simulink model "SOLARPV_BATTERY_HYBRID"  (R2023b)
settings: Solver=ode23t  StartTime=0.0  StopTime=5  FixedStep=1e-5  MaxStep=1e-4  RelTol=10e-4  EnableMultiTasking=on
undefined symbols (not defined in the file): Ion, Lithium
libraries: spsFirstOrderFilterLib x8, spsSeriesRLCBranchLib x7, simulink x7, spsCurrentMeasurementLib x4, spsPWMGeneratorDCDCLib x3, spsVoltageMeasurementLib x3, spsIGBTDiodeLib x3, slpidlib x2, spsGroundLib x2, spsPermanentMagnetSynchronousMachineLib x1, spsUniversalBridgeLib x1, spsBatteryLib x1
settings Model: Creator=Administrator  LastModifiedBy=NADIN
settings SolverCC: ZeroCrossControl=DisableAll  AlgebraicLoopSolver=TrustRegion
settings DataIOCC: LimitDataPoints=on  SaveFormat=Array  SignalLoggingSaveFormat=ModelDataLogs  ReturnWorkspaceOutputs=off
settings OptimizationCC: ExpressionDepthLimit=2147483647  LifeSpan=inf
settings DebuggingCC: UnderspecifiedInitializationDetection=Classic  MergeDetectMultiDrivingBlocksExec=none  SolverPrmCheckMsg=warning  FcnCallInpInsideContextMsg=warning  UnconnectedInputMsg=warning  UnconnectedOutputMsg=warning  UnconnectedLineMsg=warning  StateNameClashWarn=warning  SFUnexpectedBacktrackingDiag=warning  SFNoUnconditionalDefaultTransitionDiag=warning  SFExecutionAtInitializationDiag=none  ArithmeticOperatorsInVariantConditions=warning
settings HardwareCC: ProdBitPerPointer=32  ProdBitPerSizeT=32  ProdBitPerPtrDiffT=32  ProdLargestAtomicFloat=None  ProdIntDivRoundTo=Undefined  ProdEndianess=Unspecified  ProdWordSize=32  ProdHWDeviceType=32-bit Generic
settings ModelReferenceCC: EnableRefExpFcnMdlSchedulingChecks=on  PropagateSignalLabelsOutOfModel=off
settings SFSimCC: SimUseLocalCustomCode=off  CustomCodeUndefinedFunction=UseInterfaceOnly
settings RTWCC: RTWUseLocalCustomCode=off
settings CodeAppCC: StateflowObjectComments=on
settings GRTTargetCC: TargetLangStandard=C89/C90 (ANSI)  CombineOutputUpdateFcns=off  GRTInterface=on
settings ConfigComp: CovMetricSettings=dw  CovSaveCumulativeToWorkspaceVar=on  CovSaveSingleToWorkspaceVar=on  CovExternalEMLEnable=off
settings SimscapeCC: SimscapeNormalizeSystem=off

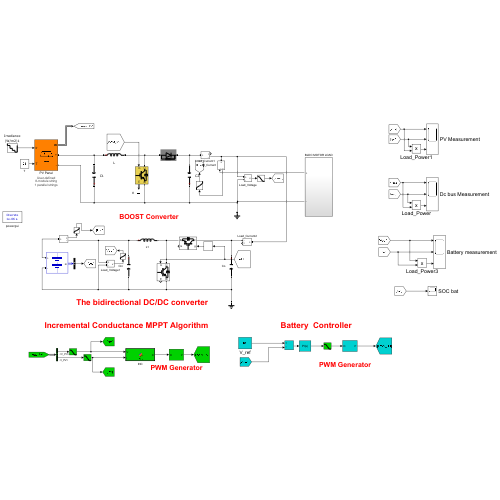
[thumbnail: Simulink's stored preview of the top-level diagram]
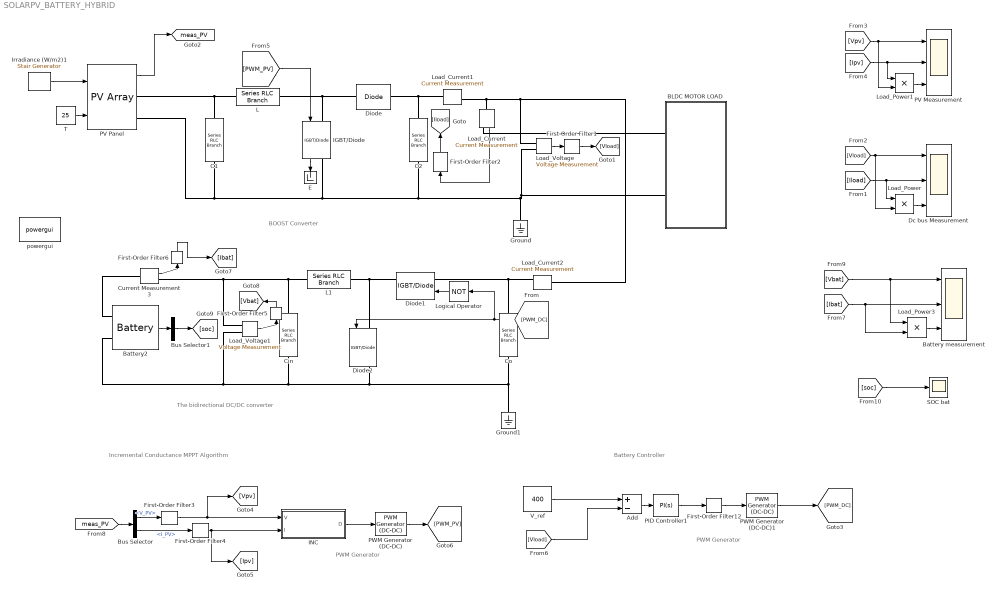
== system SOLARPV_BATTERY_HYBRID ==
  note: BOOST Converter
  note: Incremental Conductance MPPT Algorithm
  note: PWM Generator
  note: The bidirectional DC/DC converter
  note: PWM Generator
  note: Battery Controller
  Add : Sum  Inputs=+-
  BLDC MOTOR LOAD : Subsystem
  Battery measurement : Scope  NumInputPorts=3
  Battery2 : spsBatteryLib/Battery  BatType=Lithium-Ion  ShowTempParam=off  ThermalPreset=no  ShowAgeParam=off  NomV=12*20  NomQ=48  SOC=50  Batt_Tr=0.0001  PresetModel=on  MaxQ=48  MinV=180  FullV=279.3569  Dis_rate=20.8696  R=0.05  Normal_OP=43.4087  expZone="[259.2926      2.358261]"  current=[1.5 3]  Units=Ampere-hour  Tci=20  NomT=20  T2=-30  MaxQ2=4.8  FullV2=7.1  Normal_OP2=5.72  expZone2="[6.58  1]"  Rca=0.6  ti=1000  Dp=0  Neq0=0  Tsim=1e6  Ta1=25  Qeol=5.4*0.9  Reol=0.013333*1.2  Char_age=[2.3478, 3]  Dis_age=[2.3478, 10]  N1=1500  N2=10500  N3=1000  N4=1400  Ta2=45  N5=950
      settings: LibrarySourceBlock=electricdrivelib/Extra Sources/Battery
  Bus Selector : BusSelector  OutputSignals=V_PV,I_PV
  Bus Selector1 : BusSelector  OutputSignals=SOC (%)  OutputAsBus=on
  C1 : spsSeriesRLCBranchLib/Series RLC Branch  LConnTagsString=__new0  RConnTagsString=__new0  BranchType=C  Resistance=1  Inductance=1e-3  SetiL0=off  InitialCurrent=0  Capacitance=4.8250e-05  Setx0=off  InitialVoltage=0  Measurements=None
  C2 : spsSeriesRLCBranchLib/Series RLC Branch  LConnTagsString=__new0  RConnTagsString=__new0  BranchType=C  Resistance=1  Inductance=1e-3  SetiL0=off  InitialCurrent=0  Capacitance=4.8250e-05  Setx0=off  InitialVoltage=0  Measurements=None
  Cin : spsSeriesRLCBranchLib/Series RLC Branch  LConnTagsString=__new0  RConnTagsString=__new0  BranchType=C  Resistance=1  Inductance=3e-3  SetiL0=off  InitialCurrent=0  Capacitance=4.8250e-05  Setx0=off  InitialVoltage=0  Measurements=None
  Co : spsSeriesRLCBranchLib/Series RLC Branch  LConnTagsString=__new0  RConnTagsString=__new0  BranchType=C  Resistance=1  Inductance=3e-3  SetiL0=off  InitialCurrent=0  Capacitance=4.8250e-05  Setx0=off  InitialVoltage=0  Measurements=None
  Current Measurement3 : spsCurrentMeasurementLib/Current Measurement  PhasorSimulation=off  OutputType=Complex  PSBequivalent=0
  Dc bus Measurement : Scope  NumInputPorts=3
  Diode : spsDiodeLib/Diode  Ron=0.001  Lon=0  Vf=0.8  IC=0  UseSnubber=off  Rs=500  Cs=250e-9  Measurements=off
  Diode1 : spsIGBTDiodeLib/IGBT//Diode  Ron=1e-3  Rs=1e5  Cs=inf  Measurements=on
  Diode2 : spsIGBTDiodeLib/IGBT//Diode  Ron=1e-3  Rs=1e5  Cs=inf  Measurements=on
  E : Terminator
  First-Order Filter{1..6,12} (7 alike) : spsFirstOrderFilterLib/First-Order Filter  FilterType=Lowpass  Tc=10e-3  Ts=0  Initialize=on  Vac_Init=[0, 0, 60]  Vdc_Init=0  PlotResponse=off  FreqRange="[0,  200,  1]"
  Ground : spsGroundLib/Ground  LConnTagsString=a
  Ground1 : spsGroundLib/Ground  LConnTagsString=a
  IGBT/Diode : spsIGBTDiodeLib/IGBT//Diode  Ron=1e-3  Rs=1e5  Cs=inf  Measurements=on
  INC : MATLAB Function  TreatAsAtomicUnit=on
  Irradiance (W/m2)1 : spsStairGeneratorLib/Stair Generator  t=[0, 0.3, 0.6,0.9, 1.2,1.5]*(1/0.3)  e=[1, 0.8, 0.5, 0.3, 0.1,0.8]*1000  Ts=0.0001
  L : spsSeriesRLCBranchLib/Series RLC Branch  LConnTagsString=__new0  RConnTagsString=__new0  BranchType=L  Resistance=1  Inductance=0.1164  SetiL0=off  InitialCurrent=0  Capacitance=1e-6  Setx0=off  InitialVoltage=0  Measurements=None
  L1 : spsSeriesRLCBranchLib/Series RLC Branch  LConnTagsString=__new0  RConnTagsString=__new0  BranchType=L  Resistance=.25  Inductance=0.1164  SetiL0=off  InitialCurrent=0  Capacitance=1e-6  Setx0=off  InitialVoltage=0  Measurements=None
  Load_Current : spsCurrentMeasurementLib/Current Measurement  PhasorSimulation=off  OutputType=Complex  PSBequivalent=0
  Load_Current1 : spsCurrentMeasurementLib/Current Measurement  PhasorSimulation=off  OutputType=Complex  PSBequivalent=0
  Load_Current2 : spsCurrentMeasurementLib/Current Measurement  PhasorSimulation=off  OutputType=Complex  PSBequivalent=0
  Load_Power : Product  RndMeth=Zero
  Load_Power1 : Product  RndMeth=Zero
  Load_Power3 : Product  RndMeth=Zero
  Load_Voltage : spsVoltageMeasurementLib/Voltage Measurement  PhasorSimulation=off  OutputType=Complex  PSBequivalent=0
  Load_Voltage1 : spsVoltageMeasurementLib/Voltage Measurement  PhasorSimulation=off  OutputType=Complex  PSBequivalent=0
  Logical Operator : Logic  Operator=NOT  AllPortsSameDT=off  OutDataTypeStr=boolean
  PID Controller1 : slpidlib/PID Controller  Controller=PI  Form=Parallel  TimeDomain=Continuous-time  UseExternalTs=off  SampleTime=-1  IntegratorMethod=Forward Euler  FilterMethod=Forward Euler  ControllerParametersSource=internal  P=0.0001  I=0.02  UseKiTs=off  D=0  N=100  UseFilter=on  TunerSelectOption=Transfer Function Based (PID Tuner App)  InitialConditionSource=internal  InitialConditionForIntegrator=0  InitialConditionForFilter=0  DifferentiatorICPrevScaledInput=0  ExternalReset=none  TrackingMode=off  Kt=1  LimitOutput=off  SatLimitsSource=internal  UpperSaturationLimit=inf  LowerSaturationLimit=-inf  LinearizeAsGain=on  AntiWindupMode=none  Kb=1  LimitIntegrator=off  UpperIntegratorSaturationLimit=inf  LowerIntegratorSaturationLimit=-inf  POutMin=[]  POutMax=[]  IOutMin=[]  IOutMax=[]  DOutMin=[]  DOutMax=[]  NOutMin=[]  NOutMax=[]  SumOutMin=[]  SumOutMax=[]  SaturationOutMin=[]  SaturationOutMax=[]  PParamMin=[]  PParamMax=[]  IParamMin=[]  IParamMax=[]  DParamMin=[]  DParamMax=[]  NParamMin=[]  NParamMax=[]  KbParamMin=[]  KbParamMax=[]  KtParamMin=[]  KtParamMax=[]  KbOutMin=[]  KbOutMax=[]  KtOutMin=[]  KtOutMax=[]  IntegratorOutMin=[]  IntegratorOutMax=[]  FilterOutMin=[]  FilterOutMax=[]  SumI1OutMin=[]  SumI1OutMax=[]  SumI2OutMin=[]  SumI2OutMax=[]  SumI3OutMin=[]  SumI3OutMax=[]  SumI4OutMin=[]  SumI4OutMax=[]  SumDOutMin=[]  SumDOutMax=[]  DifferentiatorOutMin=[]  DifferentiatorOutMax=[]  FilterDiffOutCoefMin=[]  FilterDiffOutCoefMax=[]  ReciprocalOutMin=[]  ReciprocalOutMax=[]  SumDenOutMin=[]  SumDenOutMax=[]  SumNumOutMin=[]  SumNumOutMax=[]  DivideOutMin=[]  DivideOutMax=[]  UdiffTsProdOutMin=[]  UdiffTsProdOutMax=[]  NTsProdOutMin=[]  NTsProdOutMax=[]  UintegralTsProdOutMin=[]  UintegralTsProdOutMax=[]  UngainTsProdOutMin=[]  UngainTsProdOutMax=[]  ClampingZeroOutDataTypeStr=Inherit: Inherit via back propagation  ClampingZeroOutMin=[]  ClampingZeroOutMax=[]  FilterDenConstantOutDataTypeStr=Inherit: Inherit via back propagation  FilterDenConstantOutMin=[]  FilterDenConstantOutMax=[]  PCopyOutDataTypeStr=Inherit: Inherit via back propagation  PCopyOutMin=[]  PCopyOutMax=[]  NCopyOutDataTypeStr=Inherit: Inherit via back propagation  NCopyOutMin=[]  NCopyOutMax=[]  IntegratorContinuousStateAttributes=''  IntegratorStateMustResolveToSignalObject=off  IntegratorRTWStateStorageClass=Auto  FilterContinuousStateAttributes=''  FilterStateMustResolveToSignalObject=off  FilterRTWStateStorageClass=Auto  ParallelPVariant=InternalParameters  IdealPVariant=Disabled  IVariant=InternalParameters  DVariant=Disabled  IntegratorVariant=Continuous  SatVariant=Disabled  AWVariant=Passthrough  PCopyVariant=Disabled  TRVariant=Disabled  FdbkBlocksVariant=Forward  IdealPFdbkVariant=Disabled  SatFdbkVariant=Disabled  DerivativeFilterVariant=Disabled  NVariant=Disabled  NCopyVariant=Disabled_SignalSpec  FilterICVariant=Disabled  IntegratorICVariant=InternalICs  ExternalResetVariant=Disabled  TRSumVariant=Passthrough  SumFdbkVariant=Disabled  SumVariant=Sum_PI  TsampFilterVariant=InternalTs  TsampNgainVariant=Passthrough  TsampIntegralVariant=Disabled_SignalSpec  ExternalSaturationOutDataTypeStr=Inherit: Same as second input
  PV Measurement : Scope  NumInputPorts=3
  PV Panel : spsPVArrayLib/PV Array  Npar=1  Nser=8  PlotType=array @ 25 deg.C & specified irradiances  S_vec="[ 1000 800  600  400 ]"  Temp_C_vec="[ 45 25  ]"  ModuleName=User-defined  PlotWhenSelected=off  Pm=250.205  Ncell=60  Voc=37.3  Isc=8.66  Vm=30.7  Im=8.15  beta_Voc_pc=-0.36901  alpha_Isc_pc=0.086998  beta_Voc=-0.13764  alpha_Isc=0.007534  IL=8.7062  I0=4.1579e-10  nI=1.0189  Rsh=240.6015  Rs=0.23732  RobustModel=off  RobustCellTemperature=313.3991  BAL=on  Tc=1e-6  Tfilter=1e-5
      settings: AttributesFormatString=|
      | %<ModuleName>
      | %<Nser>-module string
      | %<Npar> parallel strings
  PWM Generator (DC-DC) : spsPWMGeneratorDCDCLib/PWM Generator (DC-DC)  Fsw=10000  Ts=0
  PWM Generator (DC-DC)1 : spsPWMGeneratorDCDCLib/PWM Generator (DC-DC)  Fsw=10000  Ts=0
  SOC bat : Scope
  T : Constant  Value=25
  V_ref : Constant  Value=400
  powergui : sps_lib/powergui  Priority=1  SimulationMode=Discrete  SampleTime=1e-6  frequency=60  Iterations=50  frequencyindice=0  Pbase=100e6  ErrMax=1e-4  UnitsV=kV  UnitsW=MW  buscounter=0  FunctionMessages=off  echomessages=off  EnableUseOfTLC=off  CurrentSourceSwitches=off  DisableSnubberDevices=off  DisableRonSwitches=off  DisableVfSwitches=off  DisplayEquations=off  AutomaticDiscreteSolvers=off  SolverType=Tustin/Backward Euler (TBE)  Interpol=off  ExternalGateDelay=off  methode=off  Ts=100  x0status=blocks  SPID=on  SwTol=0  HookPort=off  NonlinearTolerance=1e-4  nMaxIteration=100  ContinueOnMaxIteration=off  RestoreLinks=warning  ResistiveCurrentMeasurement=off  Frange=[0:2:500]  Ylog=off  Xlog=on  ShowGrid=off  save=off  variable=ZData  structure=0  ZoomFFT=off  StartTime=0.0  cycles=1  DisplayStyle=1  fundamental=60  FreqAxis=off  MaxFrequency=1000  frequencyindicesteady=1  RmsSteady=1  display=off
  tag scope: meas_PV=global
  wires:
  T/1 -> PV Panel/2
  IGBT/Diode/1 -> E/1
  PV Panel/1 -> [meas_PV]
  [meas_PV] -> Bus Selector/1
  Bus Selector/2 -> First-Order Filter4/1  "<I_PV>"
  Bus Selector/1 -> First-Order Filter3/1  "<V_PV>"
  INC/1(D) -> PWM Generator (DC-DC)/1
  V_ref/1 -> Add/1
  [Vload] -> Add/2
  Load_Voltage/1 -> First-Order Filter1/1
  Load_Current/1 -> First-Order Filter2/1
  First-Order Filter3/1 -> [Vpv], INC/1(V)
  First-Order Filter4/1 -> [Ipv], INC/2(I)
  Battery2/1 -> Bus Selector1/1
  Logical Operator/1 -> Diode1/1
  First-Order Filter2/1 -> [Iload]
  First-Order Filter1/1 -> [Vload]
  PWM Generator (DC-DC)/1 -> [PWM_PV]
  [PWM_PV] -> IGBT/Diode/1
  PWM Generator (DC-DC)1/1 -> [PWM_DC]
  [PWM_DC] -> Logical Operator/1, Diode2/1
  Current Measurement3/1 -> First-Order Filter6/1
  Load_Voltage1/1 -> First-Order Filter5/1
  Bus Selector1/1 -> [soc]
  [Vpv] -> Load_Power1/2, PV Measurement/1
  [Ipv] -> Load_Power1/1, PV Measurement/2
  Load_Power1/1 -> PV Measurement/3
  [Ibat] -> Load_Power3/2, Battery measurement/2
  [Vbat] -> Load_Power3/1, Battery measurement/1
  First-Order Filter6/1 -> [Ibat]
  First-Order Filter5/1 -> [Vbat]
  [Vload] -> Load_Power/2, Dc bus Measurement/1
  [Iload] -> Load_Power/1, Dc bus Measurement/2
  Load_Power/1 -> Dc bus Measurement/3
  [soc] -> SOC bat/1
  Load_Power3/1 -> Battery measurement/3
  PID Controller1/1 -> First-Order Filter12/1
  Add/1 -> PID Controller1/1
  First-Order Filter12/1 -> PWM Generator (DC-DC)1/1
  Irradiance (W/m2)1/1 -> PV Panel/1
  connections:
  L/LConn1 -- PV Panel/RConn1 -- C1/RConn1
  L/RConn1 -- Diode/LConn1 -- IGBT/Diode/LConn1
  Load_Voltage/LConn2 -- PV Panel/RConn2 -- C1/LConn1 -- IGBT/Diode/RConn1 -- C2/LConn1 -- Ground/LConn1 -- BLDC MOTOR LOAD/RConn2
  Diode/RConn1 -- Load_Current1/LConn1 -- C2/RConn1
  Current Measurement3/LConn1 -- Battery2/LConn1
  Load_Voltage1/LConn1 -- Current Measurement3/RConn1 -- L1/LConn1 -- Cin/LConn1
  Diode2/LConn1 -- Diode1/RConn1 -- L1/RConn1
  BLDC MOTOR LOAD/RConn1 -- Load_Current/RConn1
  Co/RConn1 -- Ground1/LConn1 -- Load_Voltage1/LConn2 -- Battery2/LConn2 -- Cin/RConn1 -- Diode2/RConn1
  Co/LConn1 -- Load_Current2/RConn1 -- Diode1/LConn1
  Load_Current1/RConn1 -- Load_Current2/LConn1 -- Load_Voltage/LConn1 -- Load_Current/LConn1

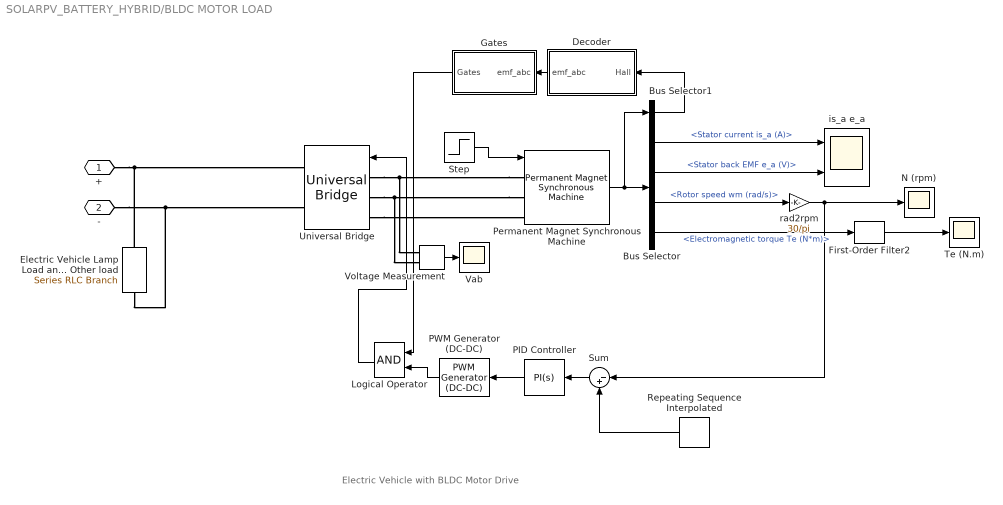
== system SOLARPV_BATTERY_HYBRID/BLDC MOTOR LOAD ==
  note: Electric Vehicle with BLDC Motor Drive
  Bus Selector : BusSelector  OutputSignals=Stator current is_a (A),Stator back EMF e_a (V),Rotor speed wm (rad/s),Electromagnetic torque Te (N*m)
  Bus Selector1 : BusSelector  OutputSignals=Hall effect signal h_a,Hall effect signal h_b,Hall effect signal h_c  OutputAsBus=on
  Decoder : Subsystem
  Electric Vehicle Lamp Load and Other load : spsSeriesRLCBranchLib/Series RLC Branch  LConnTagsString=__new0  RConnTagsString=__new0  BranchType=R  Resistance=400*400/1000  Inductance=1e-3  SetiL0=off  InitialCurrent=0  Capacitance=1e-6  Setx0=off  InitialVoltage=0  Measurements=None
  First-Order Filter2 : spsFirstOrderFilterLib/First-Order Filter  FilterType=Lowpass  Tc=10e-3  Ts=0  Initialize=on  Vac_Init=[0, 0, 60]  Vdc_Init=0  PlotResponse=off  FreqRange="[0,  200,  1]"
  Gates : Subsystem
  Logical Operator : Logic  AllPortsSameDT=off  OutDataTypeStr=boolean
  N (rpm) : Scope
  PID Controller : slpidlib/PID Controller  Controller=PI  Form=Parallel  TimeDomain=Continuous-time  UseExternalTs=off  SampleTime=-1  IntegratorMethod=Forward Euler  FilterMethod=Forward Euler  ControllerParametersSource=internal  P=1  I=1  UseKiTs=off  D=0  N=100  UseFilter=on  TunerSelectOption=Transfer Function Based (PID Tuner App)  InitialConditionSource=internal  InitialConditionForIntegrator=0  InitialConditionForFilter=0  DifferentiatorICPrevScaledInput=0  ExternalReset=none  TrackingMode=off  Kt=1  LimitOutput=off  SatLimitsSource=internal  UpperSaturationLimit=inf  LowerSaturationLimit=-inf  LinearizeAsGain=on  AntiWindupMode=none  Kb=1  LimitIntegrator=off  UpperIntegratorSaturationLimit=inf  LowerIntegratorSaturationLimit=-inf  POutMin=[]  POutMax=[]  IOutMin=[]  IOutMax=[]  DOutMin=[]  DOutMax=[]  NOutMin=[]  NOutMax=[]  SumOutMin=[]  SumOutMax=[]  SaturationOutMin=[]  SaturationOutMax=[]  PParamMin=[]  PParamMax=[]  IParamMin=[]  IParamMax=[]  DParamMin=[]  DParamMax=[]  NParamMin=[]  NParamMax=[]  KbParamMin=[]  KbParamMax=[]  KtParamMin=[]  KtParamMax=[]  KbOutMin=[]  KbOutMax=[]  KtOutMin=[]  KtOutMax=[]  IntegratorOutMin=[]  IntegratorOutMax=[]  FilterOutMin=[]  FilterOutMax=[]  SumI1OutMin=[]  SumI1OutMax=[]  SumI2OutMin=[]  SumI2OutMax=[]  SumI3OutMin=[]  SumI3OutMax=[]  SumI4OutMin=[]  SumI4OutMax=[]  SumDOutMin=[]  SumDOutMax=[]  DifferentiatorOutMin=[]  DifferentiatorOutMax=[]  FilterDiffOutCoefMin=[]  FilterDiffOutCoefMax=[]  ReciprocalOutMin=[]  ReciprocalOutMax=[]  SumDenOutMin=[]  SumDenOutMax=[]  SumNumOutMin=[]  SumNumOutMax=[]  DivideOutMin=[]  DivideOutMax=[]  UdiffTsProdOutMin=[]  UdiffTsProdOutMax=[]  NTsProdOutMin=[]  NTsProdOutMax=[]  UintegralTsProdOutMin=[]  UintegralTsProdOutMax=[]  UngainTsProdOutMin=[]  UngainTsProdOutMax=[]  ClampingZeroOutDataTypeStr=Inherit: Inherit via back propagation  ClampingZeroOutMin=[]  ClampingZeroOutMax=[]  FilterDenConstantOutDataTypeStr=Inherit: Inherit via back propagation  FilterDenConstantOutMin=[]  FilterDenConstantOutMax=[]  PCopyOutDataTypeStr=Inherit: Inherit via back propagation  PCopyOutMin=[]  PCopyOutMax=[]  NCopyOutDataTypeStr=Inherit: Inherit via back propagation  NCopyOutMin=[]  NCopyOutMax=[]  IntegratorContinuousStateAttributes=''  IntegratorStateMustResolveToSignalObject=off  IntegratorRTWStateStorageClass=Auto  FilterContinuousStateAttributes=''  FilterStateMustResolveToSignalObject=off  FilterRTWStateStorageClass=Auto  ParallelPVariant=InternalParameters  IdealPVariant=Disabled  IVariant=InternalParameters  DVariant=Disabled  IntegratorVariant=Continuous  SatVariant=Disabled  AWVariant=Passthrough  PCopyVariant=Disabled  TRVariant=Disabled  FdbkBlocksVariant=Forward  IdealPFdbkVariant=Disabled  SatFdbkVariant=Disabled  DerivativeFilterVariant=Disabled  NVariant=Disabled  NCopyVariant=Disabled_SignalSpec  FilterICVariant=Disabled  IntegratorICVariant=InternalICs  ExternalResetVariant=Disabled  TRSumVariant=Passthrough  SumFdbkVariant=Disabled  SumVariant=Sum_PI  TsampFilterVariant=InternalTs  TsampNgainVariant=Passthrough  TsampIntegralVariant=Disabled_SignalSpec  ExternalSaturationOutDataTypeStr=Inherit: Same as second input
  PWM Generator (DC-DC) : spsPWMGeneratorDCDCLib/PWM Generator (DC-DC)  Fsw=5000  Ts=0
  Permanent Magnet Synchronous Machine : spsPermanentMagnetSynchronousMachineLib/Permanent Magnet Synchronous Machine  NbPhases=3  FluxDistribution=Trapezoidal  RotorType=Round  MechanicalLoad=Torque Tm  PresetModel=No  ShowDetailedParameters=on  MeasurementBus=off  Resistance=2.8750  Inductance=8.5e-3  dqInductances=[8.5e-3, 8.5e-3]  La=0.000835  MachineConstant=Flux linkage established by magnets (V.s)  Flux=0.175  VoltageCst=146.6077  TorqueCst=1.4  Flat=120  Mechanical=[ 0.8e-3, 1e-3 4]  PolePairs=4  InitialConditions=[0,0, 0,0]  InitialConditions5ph=[0 0 0 0 0 0]  RefAngle=90 degrees behind phase A axis (modified Park)  IterativeDiscreteModel=Trapezoidal non iterative  TsBlock=-1  TsPowergui=0
  Repeating Sequence Interpolated : simulink/Sources/Repeating Sequence Interpolated  OutValues=[0 2000 2000 0].'  TimeValues=[0 1.5 3.5 5].'  LookUpMeth=Interpolation-Use End Values  tsamp=0.01  OutMin=[]  OutMax=[]  OutDataTypeStr=double  OutputDataTypeScalingMode=double  OutDataType=fixdt(0,8)  OutScaling=2^-10
  Step : Step  Time=.1  Before=3  After=3  SampleTime=0
  Sum : Sum  Inputs=|-+
  Te (N.m) : Scope
  Universal Bridge : spsUniversalBridgeLib/Universal Bridge  Arms=3  SnubberResistance=5000  SnubberCapacitance=1e-6  Device=MOSFET / Diodes  Ron=1e-3  Lon=0  ForwardVoltages="[  0  0  ]"  ForwardVoltage=0  GTOparameters=[ 10e-6 , 20e-6 ]  IGBTparameters=[ 1e-6 , 2e-6 ]  Measurements=None  Measurements_2=None  converterType=Rectifier
  Vab : Scope
  Voltage Measurement : spsVoltageMeasurementLib/Voltage Measurement  PhasorSimulation=off  OutputType=Complex  PSBequivalent=0
  is_a e_a : Scope  NumInputPorts=2
  rad2rpm : Gain  Gain=30/pi
  + : PMIOPort  Side=Right
  - : PMIOPort  Port=2  Side=Right
  wires:
  Voltage Measurement/1 -> Vab/1
  Step/1 -> Permanent Magnet Synchronous Machine/1
  Decoder/1(emf_abc) -> Gates/1("emf_abc ")
  rad2rpm/1 -> Sum/1, N (rpm)/1
  Bus Selector/2 -> is_a e_a/2  "<Stator back EMF e_a (V)>"
  Bus Selector1/1 -> Decoder/1("Hall ")
  Bus Selector/1 -> is_a e_a/1  "<Stator current is_a (A)>"
  Bus Selector/3 -> rad2rpm/1  "<Rotor speed wm (rad/s)>"
  Bus Selector/4 -> First-Order Filter2/1  "<Electromagnetic torque Te (N*m)>"
  Permanent Magnet Synchronous Machine/1 -> Bus Selector/1, Bus Selector1/1
  Sum/1 -> PID Controller/1
  PID Controller/1 -> PWM Generator (DC-DC)/1
  PWM Generator (DC-DC)/1 -> Logical Operator/2
  Gates/1(Gates) -> Logical Operator/1
  Logical Operator/1 -> Universal Bridge/1
  Repeating Sequence Interpolated/1 -> Sum/2
  First-Order Filter2/1 -> Te (N.m)/1
  connections:
  -/RConn1 -- Electric Vehicle Lamp Load and Other load/RConn1 -- Universal Bridge/RConn2
  Universal Bridge/LConn3 -- Permanent Magnet Synchronous Machine/LConn3
  +/RConn1 -- Electric Vehicle Lamp Load and Other load/LConn1 -- Universal Bridge/RConn1
  Permanent Magnet Synchronous Machine/LConn2 -- Universal Bridge/LConn2 -- Voltage Measurement/LConn2
  Permanent Magnet Synchronous Machine/LConn1 -- Universal Bridge/LConn1 -- Voltage Measurement/LConn1

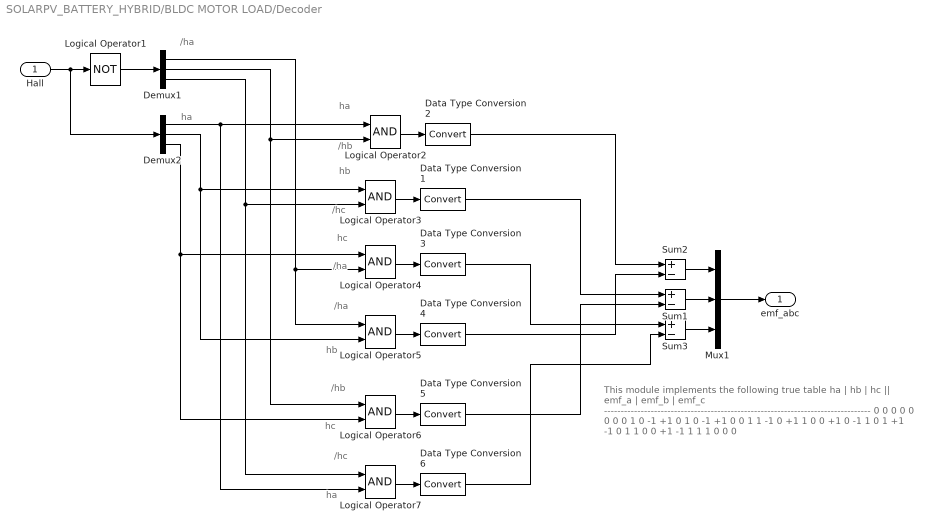
== system SOLARPV_BATTERY_HYBRID/BLDC MOTOR LOAD/Decoder ==
  note: /ha
  note: ha
  note: ha
  note: /hb
  note: hb
  note: /hc
  note: hc
  note: /ha
  note: /ha
  note: hb
  note: /hb
  note: hc
  note: /hc
  note: ha
  note: This module implements the following true table
      |
      |    ha   |   hb   |   hc   ||   emf_a   |   emf_b   |   emf_c
      |     --------------------------------------------------------------------------------
      | 0          0         0          0               0               0
      | 0          0         1          0               -1              +1
      | 0          1         0          -1              +1                0
      | 0          1         1          -1               0               +1
      | 1          0         0         +1               0               -1
      | 1          0         1         +1              -1                0
      | 1          1         0          0              +1               -1
      | 1          1         1          0               0                0
  "Hall " : Inport
  Data Type Conversion{1..6} (6 alike) : DataTypeConversion  SaturateOnIntegerOverflow=off  RndMeth=Floor
  Demux1 : Demux  Outputs=3
  Demux2 : Demux  Outputs=3
  Logical Operator1 : Logic  Operator=NOT  AllPortsSameDT=off  OutDataTypeStr=boolean
  Logical Operator{2..7} (6 alike) : Logic  AllPortsSameDT=off  OutDataTypeStr=boolean
  Mux1 : Mux  Inputs=3
  Sum1 : Sum  Inputs=+-  OutDataTypeStr=double
  Sum2 : Sum  Inputs=+-  OutDataTypeStr=double
  Sum3 : Sum  Inputs=+-  OutDataTypeStr=double
  emf_abc : Outport  VectorParamsAs1DForOutWhenUnconnected=off
  wires:
  "Hall "/1 -> Logical Operator1/1, Demux2/1
  Logical Operator1/1 -> Demux1/1
  Demux2/3 -> Logical Operator4/1, Logical Operator6/2
  Demux2/2 -> Logical Operator3/1, Logical Operator5/2
  Demux2/1 -> Logical Operator2/1, Logical Operator7/2
  Demux1/3 -> Logical Operator3/2, Logical Operator7/1
  Demux1/2 -> Logical Operator2/2, Logical Operator6/1
  Demux1/1 -> Logical Operator4/2, Logical Operator5/1
  Logical Operator2/1 -> Data Type Conversion2/1
  Sum2/1 -> Mux1/1
  Sum1/1 -> Mux1/2
  Sum3/1 -> Mux1/3
  Mux1/1 -> emf_abc/1
  Logical Operator3/1 -> Data Type Conversion1/1
  Logical Operator4/1 -> Data Type Conversion3/1
  Logical Operator5/1 -> Data Type Conversion4/1
  Logical Operator6/1 -> Data Type Conversion5/1
  Logical Operator7/1 -> Data Type Conversion6/1
  Data Type Conversion2/1 -> Sum2/1
  Data Type Conversion4/1 -> Sum2/2
  Data Type Conversion1/1 -> Sum1/1
  Data Type Conversion5/1 -> Sum1/2
  Data Type Conversion3/1 -> Sum3/1
  Data Type Conversion6/1 -> Sum3/2

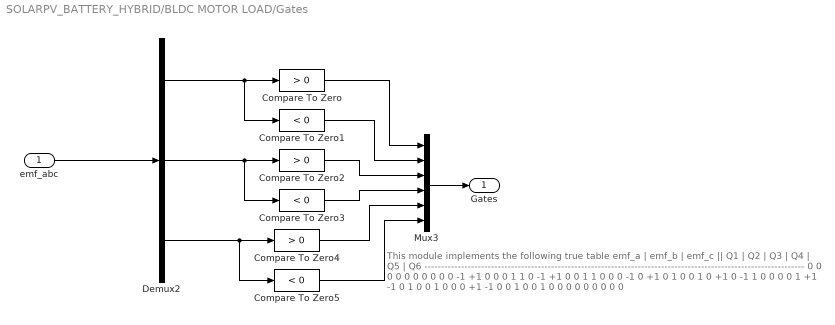
== system SOLARPV_BATTERY_HYBRID/BLDC MOTOR LOAD/Gates ==
  note: This module implements the following true table
      |
      |    emf_a   |   emf_b   |   emf_c   ||   Q1   |   Q2   |   Q3   |   Q4   |   Q5   |   Q6
      |     ------------------------------------------------------------------------------------------------------------------
      |       0              0                0            0          0          0           0        0        0
      |       0               -1              +1          0          0          0           1        1        0
      |     -1              +1                0          0          1          1           0        0        0
      |     -1               0               +1          0          1         0           0        1        0
      |    +1               0                -1          1          0          0           0        0        1
      |    +1              -1                0           1          0          0           1        0        0
      |      0              +1               -1           0          0          1           0        0        1
      |     0              0                0             0          0          0           0        0        0
  "emf_abc " : Inport
  Compare To Zero : simulink/Logic and Bit Operations/Compare To Zero  relop=>  OutDataTypeStr=boolean  ZeroCross=off
  Compare To Zero1 : simulink/Logic and Bit Operations/Compare To Zero  relop=<  OutDataTypeStr=boolean  ZeroCross=off
  Compare To Zero2 : simulink/Logic and Bit Operations/Compare To Zero  relop=>  OutDataTypeStr=boolean  ZeroCross=off
  Compare To Zero3 : simulink/Logic and Bit Operations/Compare To Zero  relop=<  OutDataTypeStr=boolean  ZeroCross=off
  Compare To Zero4 : simulink/Logic and Bit Operations/Compare To Zero  relop=>  OutDataTypeStr=boolean  ZeroCross=off
  Compare To Zero5 : simulink/Logic and Bit Operations/Compare To Zero  relop=<  OutDataTypeStr=boolean  ZeroCross=off
  Demux2 : Demux  Outputs=3
  Mux3 : Mux  Inputs=6
  Gates : Outport  VectorParamsAs1DForOutWhenUnconnected=off
  wires:
  "emf_abc "/1 -> Demux2/1
  Mux3/1 -> Gates/1
  Demux2/1 -> Compare To Zero/1, Compare To Zero1/1
  Demux2/2 -> Compare To Zero2/1, Compare To Zero3/1
  Demux2/3 -> Compare To Zero4/1, Compare To Zero5/1
  Compare To Zero/1 -> Mux3/1
  Compare To Zero1/1 -> Mux3/2
  Compare To Zero2/1 -> Mux3/3
  Compare To Zero3/1 -> Mux3/4
  Compare To Zero4/1 -> Mux3/5
  Compare To Zero5/1 -> Mux3/6

== matlab function SOLARPV_BATTERY_HYBRID/INC ==
  settings: updateMethod=DISCRETE
  data: D output; V input; I input
% author : Saad MOTAHHIR
% f= 10000hz (G)
function D  = INC(V, I)

Dinit = 0.4;  %Initial value for D output
Dmax = 0.6;   %Maximum value for D
Dmin = 0.3;   %Minimum value for D
deltaD = 0.0000005; %Increment value used to increase/decrease the duty cycle D

  
persistent Vold Pold Dold M Iold;

dataType = 'double';

if isempty(Vold)
    Vold=0;
    Pold=0;
    Iold=0;
    Dold=Dinit;
    M=1;
end
P= V*I;
dV= V - Vold;
dP= P - Pold;
dI= I - Iold;
M=1;

if M < 0.005
    D=Dold;
else
    if dV == 0
        if dI == 0
            D=Dold;
        elseif dI>0
            D=Dold - (M*deltaD);
        else 
            D=Dold + (M*deltaD);
        end    
    else
        if dI/dV == -I/V
            D=Dold;
        elseif dI/dV>-I/V    
           D=Dold - (M*deltaD);
        else
           D=Dold + (M*deltaD);  
        end  
    end    
end

if D >= Dmax | D<= Dmin
    D=Dold;
end

Dold=D;
Vold=V;
Pold=P;
Iold=I;
